simulink model "FINAL"  (R2023b)
settings: Solver=VariableStepAuto  StartTime=0.0  StopTime=50  RelTol=1e-3
libraries: spsThreePhaseParallelRLCLoadLib x4, spsThreePhaseBreakerLib x3, spsRMSLib x2, spsPower3phInstantaneousLib x1, spsThreePhasePISectionLineLib x1, spsThreePhaseVIMeasurementLib x1, spsThreePhaseSourceLib x1, sps_lib x1, spsThreePhaseTransformerTwoWindingsLib x1
settings Model: Creator=Murugaraj  LastModifiedBy=PC

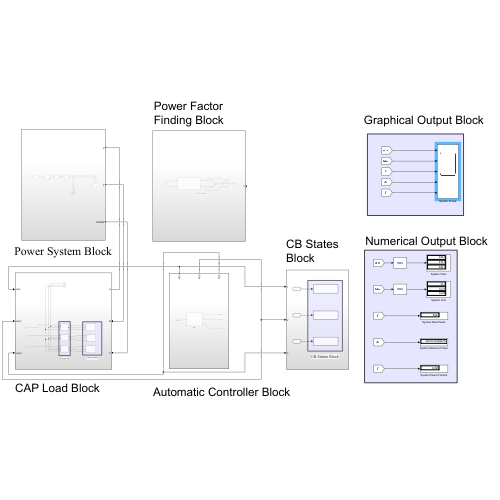
[thumbnail: Simulink's stored preview of the top-level diagram]
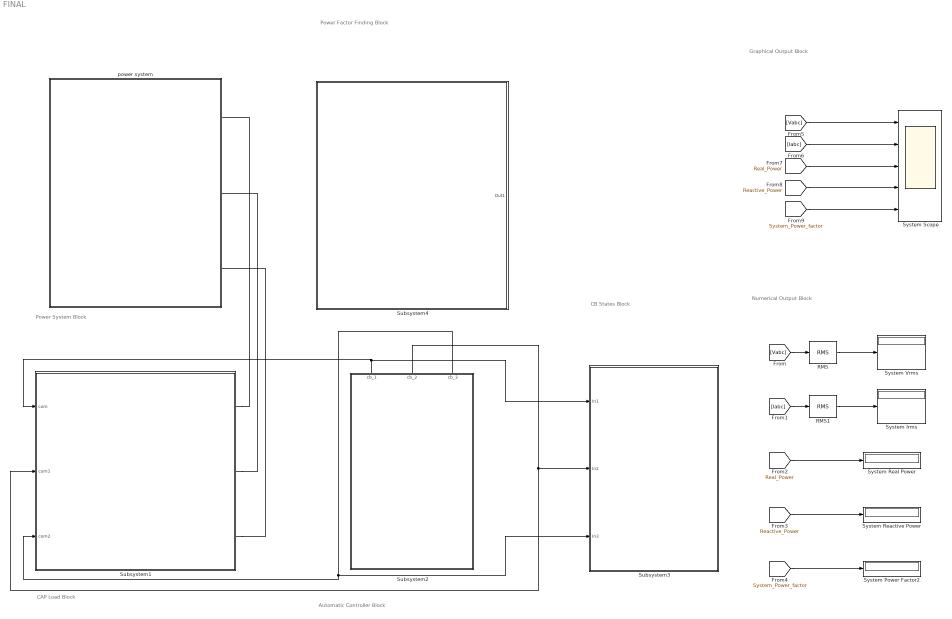
== system FINAL ==
  note: Automatic Controller Block
  note: CAP Load Block
  note: Power Factor Finding Block
  note: Power System Block
  note: Graphical Output Block
  note: Numerical Output Block
  note: CB States Block
  RMS : spsRMSLib/RMS  TrueRMS=on  Freq=60  RMSInit=120  Ts=0
  RMS1 : spsRMSLib/RMS  TrueRMS=on  Freq=60  RMSInit=120  Ts=0
  Subsystem1 : Subsystem
  Subsystem2 : Subsystem
  Subsystem3 : Subsystem
  Subsystem4 : Subsystem
  System Irms : Display
  System Power Factor2 : Display
  System Reactive Power : Display
  System Real Power : Display
  System Scope : Scope  NumInputPorts=5
  System Vrms : Display
  power system : Subsystem
  wires:
  [Vabc] -> RMS/1
  RMS/1 -> System Vrms/1
  [Iabc] -> RMS1/1
  RMS1/1 -> System Irms/1
  [Real_Power] -> System Real Power/1
  [Reactive_Power] -> System Reactive Power/1
  [System_Power_factor] -> System Power Factor2/1
  Subsystem2/1(cb_1) -> Subsystem1/1(com), Subsystem3/1(In1)
  Subsystem2/2(cb_2) -> Subsystem3/2(In2), Subsystem1/2(com1)
  Subsystem2/3(cb_3) -> Subsystem1/3(com2), Subsystem3/3(In3)
  [System_Power_factor] -> System Scope/5
  [Vabc] -> System Scope/1
  [Iabc] -> System Scope/2
  [Reactive_Power] -> System Scope/4
  [Real_Power] -> System Scope/3
  connections:
  Subsystem1/RConn1 -- power system/LConn1
  Subsystem1/RConn2 -- power system/LConn2
  Subsystem1/RConn3 -- power system/LConn3

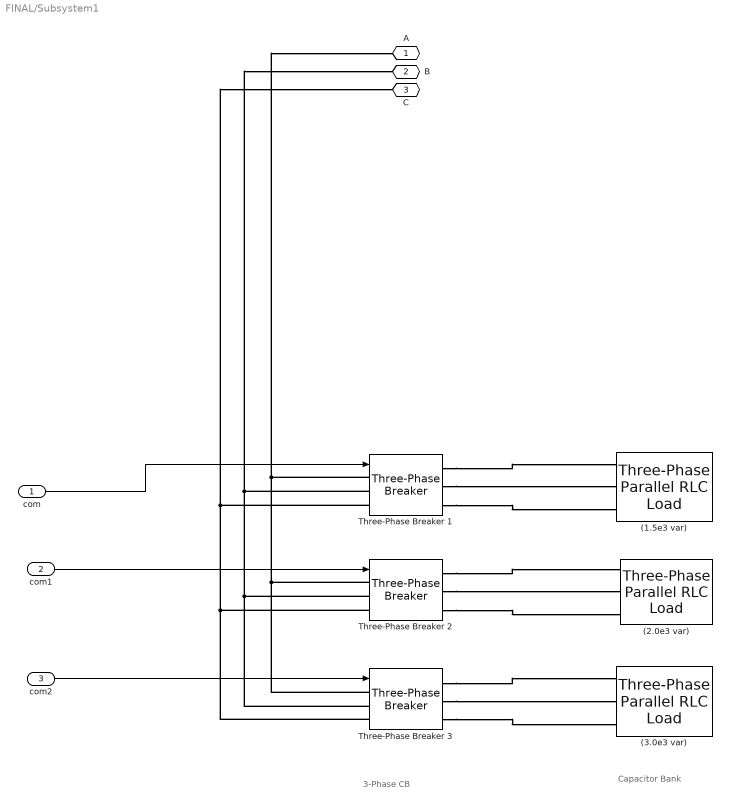
== system FINAL/Subsystem1 ==
  note: 3-Phase CB
  note: Capacitor Bank
  com : Inport
  com1 : Inport  Port=2
  com2 : Inport  Port=3
  (1.5e3 var) : spsThreePhaseParallelRLCLoadLib/Three-Phase Parallel RLC Load  LConnTagsString=A|B|C  Configuration=Y (grounded)  NominalVoltage=0.415e3  Vabc=[1e3 1e3 1e3]  Vabcp=[1e3 1e3 1e3]  NominalFrequency=50  UnbalancedPower=off  ActivePower=0  InductivePower=0  CapacitivePower=1.5e3  Pabc=[10e3 9e3 11e3]  QLabc=[100 90 110]  QCabc=[100 90 110]  Pabcp=[10e3 9e3 11e3]  QLabcp=[100 90 110]  QCabcp=[100 90 110]  Measurements=None  LoadType=constant Z
  (2.0e3 var) : spsThreePhaseParallelRLCLoadLib/Three-Phase Parallel RLC Load  LConnTagsString=A|B|C  Configuration=Y (grounded)  NominalVoltage=0.415e3  Vabc=[1e3 1e3 1e3]  Vabcp=[1e3 1e3 1e3]  NominalFrequency=50  UnbalancedPower=off  ActivePower=0  InductivePower=0  CapacitivePower=2e3  Pabc=[10e3 9e3 11e3]  QLabc=[100 90 110]  QCabc=[100 90 110]  Pabcp=[10e3 9e3 11e3]  QLabcp=[100 90 110]  QCabcp=[100 90 110]  Measurements=None  LoadType=constant Z
  (3.0e3 var) : spsThreePhaseParallelRLCLoadLib/Three-Phase Parallel RLC Load  LConnTagsString=A|B|C  Configuration=Y (grounded)  NominalVoltage=0.415e3  Vabc=[1e3 1e3 1e3]  Vabcp=[1e3 1e3 1e3]  NominalFrequency=50  UnbalancedPower=off  ActivePower=0  InductivePower=0  CapacitivePower=3e3  Pabc=[10e3 9e3 11e3]  QLabc=[100 90 110]  QCabc=[100 90 110]  Pabcp=[10e3 9e3 11e3]  QLabcp=[100 90 110]  QCabcp=[100 90 110]  Measurements=None  LoadType=constant Z
  Three-Phase Breaker 1 : spsThreePhaseBreakerLib/Three-Phase Breaker  InitialState=closed  SwitchA=on  SwitchB=on  SwitchC=on  SwitchTimes="[1/60  5/60]"  External=on  BreakerResistance=0.01  SnubberResistance=1e6  SnubberCapacitance=inf  Measurements=None
  Three-Phase Breaker 2 : spsThreePhaseBreakerLib/Three-Phase Breaker  InitialState=closed  SwitchA=on  SwitchB=on  SwitchC=on  SwitchTimes="[1/60  5/60]"  External=on  BreakerResistance=0.01  SnubberResistance=1e6  SnubberCapacitance=inf  Measurements=None
  Three-Phase Breaker 3 : spsThreePhaseBreakerLib/Three-Phase Breaker  InitialState=closed  SwitchA=on  SwitchB=on  SwitchC=on  SwitchTimes="[1/60  5/60]"  External=on  BreakerResistance=0.01  SnubberResistance=1e6  SnubberCapacitance=inf  Measurements=None
  A : PMIOPort  Side=Right
  B : PMIOPort  Port=2  Side=Right
  C : PMIOPort  Port=3  Side=Right
  wires:
  com1/1 -> Three-Phase Breaker 2/1
  com/1 -> Three-Phase Breaker 1/1
  com2/1 -> Three-Phase Breaker 3/1
  connections:
  Three-Phase Breaker 3/LConn2 -- B/RConn1 -- Three-Phase Breaker 1/LConn2 -- Three-Phase Breaker 2/LConn2
  Three-Phase Breaker 3/LConn1 -- Three-Phase Breaker 2/LConn1 -- A/RConn1 -- Three-Phase Breaker 1/LConn1
  Three-Phase Breaker 3/LConn3 -- C/RConn1 -- Three-Phase Breaker 1/LConn3 -- Three-Phase Breaker 2/LConn3
  Three-Phase Breaker 1/RConn1 -- (1.5e3 var)/LConn1
  Three-Phase Breaker 3/RConn3 -- (3.0e3 var)/LConn3
  Three-Phase Breaker 1/RConn2 -- (1.5e3 var)/LConn2
  Three-Phase Breaker 2/RConn2 -- (2.0e3 var)/LConn2
  Three-Phase Breaker 1/RConn3 -- (1.5e3 var)/LConn3
  Three-Phase Breaker 3/RConn2 -- (3.0e3 var)/LConn2
  Three-Phase Breaker 2/RConn1 -- (2.0e3 var)/LConn1
  Three-Phase Breaker 2/RConn3 -- (2.0e3 var)/LConn3
  Three-Phase Breaker 3/RConn1 -- (3.0e3 var)/LConn1

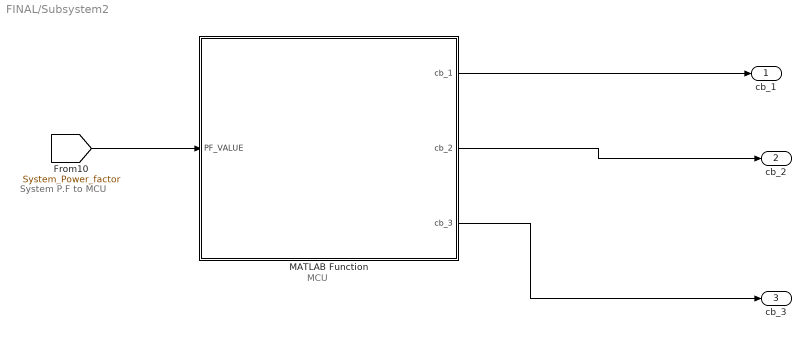
== system FINAL/Subsystem2 ==
  note: System P.F to MCU
  note: MCU
  MATLAB Function : MATLAB Function  TreatAsAtomicUnit=on
  cb_1 : Outport
  cb_2 : Outport  Port=2
  cb_3 : Outport  Port=3
  wires:
  [System_Power_factor] -> MATLAB Function/1(PF_VALUE)
  MATLAB Function/1(cb_1) -> cb_1/1
  MATLAB Function/3(cb_3) -> cb_3/1
  MATLAB Function/2(cb_2) -> cb_2/1

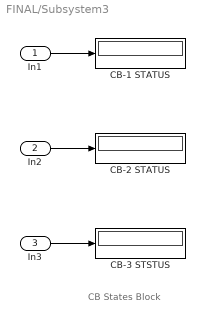
== system FINAL/Subsystem3 ==
  note: CB States Block
  In1 : Inport
  In2 : Inport  Port=2
  In3 : Inport  Port=3
  CB-1 STATUS : Display
  CB-2 STATUS : Display
  CB-3 STSTUS : Display
  wires:
  In1/1 -> CB-1 STATUS/1
  In3/1 -> CB-3 STSTUS/1
  In2/1 -> CB-2 STATUS/1

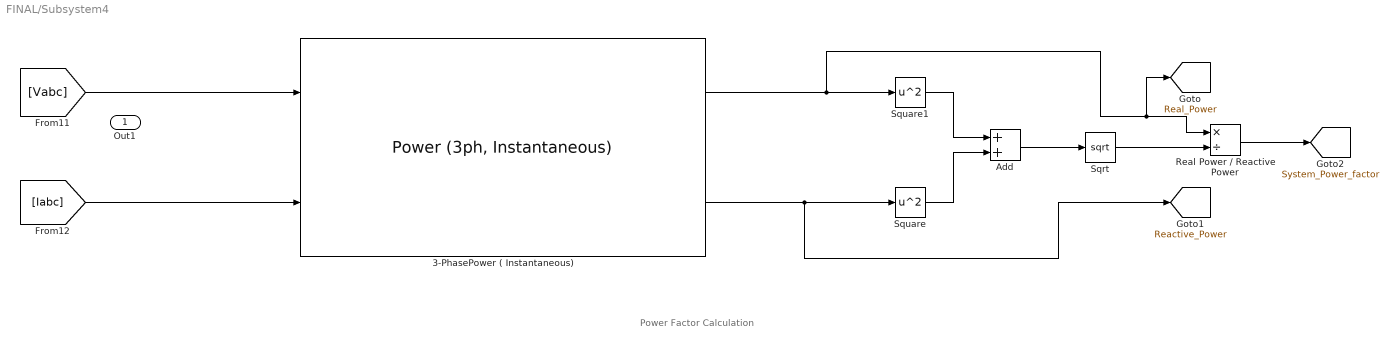
== system FINAL/Subsystem4 ==
  note: Power Factor Calculation
  3-PhasePower ( Instantaneous) : spsPower3phInstantaneousLib/Power (3ph, Instantaneous)
  Add : Sum
  Real Power / Reactive Power : Product  Inputs=*/
  Sqrt : Sqrt
  Square : Math  Operator=square
  Square1 : Math  Operator=square
  Out1 : Outport
  tag scope: Reactive_Power=global, Real_Power=global, System_Power_factor=global
  wires:
  Sqrt/1 -> Real Power / Reactive Power/2
  Real Power / Reactive Power/1 -> [System_Power_factor]
  3-PhasePower ( Instantaneous)/2 -> [Reactive_Power], Square/1
  [Iabc] -> 3-PhasePower ( Instantaneous)/2
  Square/1 -> Add/2
  Square1/1 -> Add/1
  3-PhasePower ( Instantaneous)/1 -> Real Power / Reactive Power/1, [Real_Power], Square1/1
  Add/1 -> Sqrt/1
  [Vabc] -> 3-PhasePower ( Instantaneous)/1

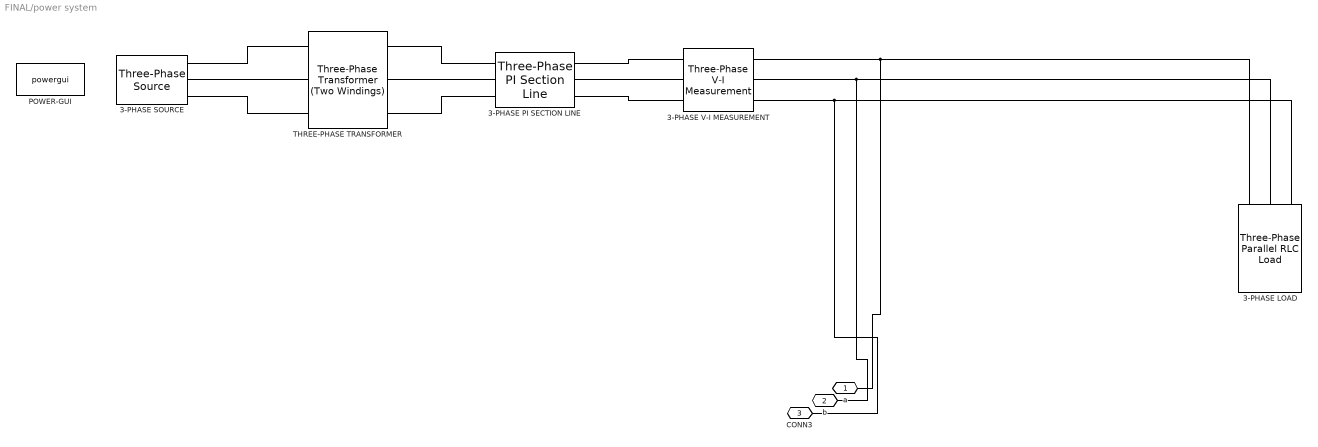
== system FINAL/power system ==
  3-PHASE PI SECTION LINE : spsThreePhasePISectionLineLib/Three-Phase PI Section Line  LConnTagsString=a|b|c  RConnTagsString=A|B|C  Length=0.01  Frequency=50  Resistances=[ 0.01273 0.3864]  Inductances="[ 0.9337e-3  4.1264e-3]"  Capacitances=[12.74e-9 7.751e-9]
  3-PHASE V-I MEASUREMENT : spsThreePhaseVIMeasurementLib/Three-Phase V-I Measurement  VoltageMeasurement=phase-to-ground  SetLabelV=on  LabelV=Vabc  Vpu=off  VpuLL=off  CurrentMeasurement=yes  SetLabelI=on  LabelI=Iabc  Ipu=off  Pbase=100e6  Vbase=500e3  OutputType=Complex  PhasorSimulation=off  PSBequivalent=0
  3-PHASE LOAD : spsThreePhaseParallelRLCLoadLib/Three-Phase Parallel RLC Load  LConnTagsString=A|B|C  Configuration=Y (grounded)  NominalVoltage=0.415e3  Vabc=[1e3 1e3 1e3]  Vabcp=[1e3 1e3 1e3]  NominalFrequency=50  UnbalancedPower=off  ActivePower=10e3  InductivePower=1e3  CapacitivePower=0  Pabc=[10e3 9e3 11e3]  QLabc=[100 90 110]  QCabc=[100 90 110]  Pabcp=[10e3 9e3 11e3]  QLabcp=[100 90 110]  QCabcp=[100 90 110]  Measurements=None  LoadType=constant Z
  3-PHASE SOURCE : spsThreePhaseSourceLib/Three-Phase Source  InternalConnection=Yg  VoltagePhases=off  Voltage=11e3  PhaseAngle=0  Voltage_phases=[25e3 25e3 25e3]/sqrt(3)  PhaseAngles_phases=[0 -120 +120]  Frequency=50  NonIdealSource=on  SpecifyImpedance=off  Resistance=0.8929  Inductance=16.58e-3  ShortCircuitLevel=100e6  BaseVoltage=25e3  XRratio=7  BusType=swing  Pref=10e3  Qref=0  Prefabc=[10e3, 10e3, 10e3]  Qrefabc=[0, 0, 0]  Qmin=-inf  Qmax=inf
  POWER-GUI : sps_lib/powergui  Priority=1  SimulationMode=Discrete  SampleTime=50e-6  frequency=60  Iterations=50  frequencyindice=0  Pbase=100e6  ErrMax=1e-4  UnitsV=kV  UnitsW=MW  buscounter=0  FunctionMessages=off  echomessages=off  EnableUseOfTLC=off  CurrentSourceSwitches=off  DisableSnubberDevices=off  DisableRonSwitches=off  DisableVfSwitches=off  DisplayEquations=off  AutomaticDiscreteSolvers=off  SolverType=Tustin/Backward Euler (TBE)  Interpol=off  ExternalGateDelay=off  methode=off  Ts=100  x0status=blocks  SPID=on  SwTol=0  HookPort=off  NonlinearTolerance=1e-4  nMaxIteration=100  ContinueOnMaxIteration=off  RestoreLinks=warning  ResistiveCurrentMeasurement=off  Frange=[0:2:500]  Ylog=off  Xlog=on  ShowGrid=off  save=off  variable=ZData  structure=0  ZoomFFT=off  StartTime=0.0  cycles=1  DisplayStyle=1  fundamental=60  FreqAxis=off  MaxFrequency=1000  frequencyindicesteady=1  RmsSteady=1  display=off
  "THREE-PHASE TRANSFORMER " : spsThreePhaseTransformerTwoWindingsLib/Three-Phase Transformer (Two Windings)  Winding1Connection=Yg  Winding2Connection=Yg  CoreType=Three single-phase transformers  SetSaturation=off  Hysteresis=off  DataFile='hysteresis'  SetInitialFlux=off  Measurements=None  UNITS=pu  NominalPower=[ 25e6 , 50 ]  Winding1=[ 11e3 , 0.002 , 0.08 ]  Winding2=[ 0.415e3 , 0.002 , 0.08 ]  Rm=500  Lm=500  L0=0.5  Saturation=[ 0,0 ; 0.0024,1.2 ; 1.0,1.52 ]  InitialFluxes=[ 0.8 , -0.8 , 0.7 ]  BreakLoop=off  DiscreteSolver=Trapezoidal iterative  DataType=off  TransfoNumber=1
  a : PMIOPort  Side=Left
  b : PMIOPort  Port=2  Side=Left
  CONN3 : PMIOPort  Port=3  Side=Left
  connections:
  3-PHASE SOURCE/RConn1 -- "THREE-PHASE TRANSFORMER "/LConn1
  3-PHASE PI SECTION LINE/RConn2 -- 3-PHASE V-I MEASUREMENT/LConn2
  3-PHASE V-I MEASUREMENT/RConn3 -- CONN3/RConn1 -- 3-PHASE LOAD/LConn3
  3-PHASE PI SECTION LINE/RConn3 -- 3-PHASE V-I MEASUREMENT/LConn3
  3-PHASE LOAD/LConn2 -- b/RConn1 -- 3-PHASE V-I MEASUREMENT/RConn2
  3-PHASE LOAD/LConn1 -- a/RConn1 -- 3-PHASE V-I MEASUREMENT/RConn1
  3-PHASE PI SECTION LINE/RConn1 -- 3-PHASE V-I MEASUREMENT/LConn1
  "THREE-PHASE TRANSFORMER "/RConn2 -- 3-PHASE PI SECTION LINE/LConn2
  3-PHASE SOURCE/RConn2 -- "THREE-PHASE TRANSFORMER "/LConn2
  "THREE-PHASE TRANSFORMER "/RConn1 -- 3-PHASE PI SECTION LINE/LConn1
  3-PHASE SOURCE/RConn3 -- "THREE-PHASE TRANSFORMER "/LConn3
  3-PHASE PI SECTION LINE/LConn3 -- "THREE-PHASE TRANSFORMER "/RConn3

== matlab function FINAL/Subsystem2/MATLAB Function ==
  data: PF_VALUE input; cb_1 output; cb_2 output; cb_3 output
function[cb_1,cb_2,cb_3] = ARDUINO_UNO(PF_VALUE)
if(PF_VALUE<=0.60)
    cb_1=1;
    cb_2=0;
    cb_3=0;
elseif(PF_VALUE<=0.75)
    cb_1=0;
    cb_2=1;
    cb_3=0;
elseif(PF_VALUE<=0.85)
    cb_1=0;
    cb_2=0;
    cb_3=1;
else
    cb_1=0;
    cb_2=0;
    cb_3=0;
    
end
